simulink model "mavsim_chap4"  (R2022b)
settings: Solver=ode45  StartTime=0.0  StopTime=10000  RelTol=1e-3  EnableMultiTasking=on
InitFcn:
  | addpath('../chap_2')
  | addpath('../../parameters/')
  | aerosonde_parameters
  | simulation_parameters
  | wind_parameters
  | addpath('../chap_3')
  | addpath('../chap_4')
  | addpath('../../tools/')
undefined symbols (not defined in the file or in its folder): drawAircraft, forces_moments, MAV, plotmavstatevariables, SIM, WIND
libraries: simulink x4
settings Model: Creator=beard  LastModifiedBy=william
settings SolverCC: AlgebraicLoopSolver=TrustRegion
settings DataIOCC: LimitDataPoints=on  SaveFormat=Array  SignalLoggingSaveFormat=ModelDataLogs  ReturnWorkspaceOutputs=off
settings OptimizationCC: ExpressionDepthLimit=2147483647  InitFltsAndDblsToZero=on  LifeSpan=inf
settings DebuggingCC: UnderspecifiedInitializationDetection=Classic  MergeDetectMultiDrivingBlocksExec=none  SolverPrmCheckMsg=warning  FcnCallInpInsideContextMsg=warning  UnconnectedInputMsg=warning  UnconnectedOutputMsg=warning  UnconnectedLineMsg=warning  StateNameClashWarn=warning  SFUnexpectedBacktrackingDiag=warning  SFNoUnconditionalDefaultTransitionDiag=warning  SFExecutionAtInitializationDiag=none  SFMachineParentedDataDiag=warning  ArithmeticOperatorsInVariantConditions=warning
settings HardwareCC: ProdBitPerPointer=32  ProdBitPerSizeT=32  ProdBitPerPtrDiffT=32  ProdLargestAtomicFloat=None  ProdIntDivRoundTo=Undefined  ProdEndianess=Unspecified  ProdWordSize=32  ProdHWDeviceType=32-bit Generic
settings ModelReferenceCC: EnableRefExpFcnMdlSchedulingChecks=on  PropagateSignalLabelsOutOfModel=off
settings SFSimCC: SimUseLocalCustomCode=off  CustomCodeUndefinedFunction=UseInterfaceOnly
settings RTWCC: RTWUseLocalCustomCode=off
settings CodeAppCC: StateflowObjectComments=on
settings GRTTargetCC: TargetLangStandard=C89/C90 (ANSI)  CombineOutputUpdateFcns=off  GRTInterface=on
settings ConfigComp: CovMetricSettings=dw  CovSaveCumulativeToWorkspaceVar=on  CovSaveSingleToWorkspaceVar=on  CovExternalEMLEnable=off  CovSFcnEnable=off

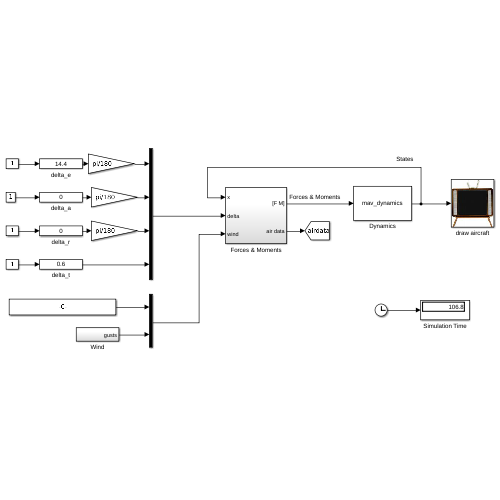
[thumbnail: Simulink's stored preview of the top-level diagram]
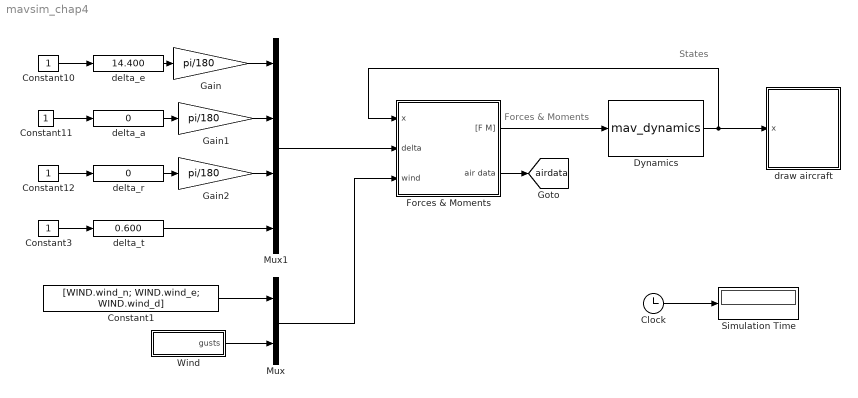
== system mavsim_chap4 ==
  note: Forces & Moments
  note: States
  Clock : Clock
  Constant1 : Constant  Value=[WIND.wind_n; WIND.wind_e; WIND.wind_d]
  Constant{3,10..12} (4 alike) : Constant
  Dynamics : S-Function  FunctionName=mav_dynamics  Parameters=MAV  SFunctionDeploymentMode=off  EnableBusSupport=off
  Forces & Moments : Subsystem
  Gain : Gain  Gain=pi/180
  Gain1 : Gain  Gain=pi/180
  Gain2 : Gain  Gain=pi/180
  Mux : Mux  Inputs=2
  Mux1 : Mux
  Simulation Time : Display
  Wind : Subsystem
  delta_a : simulink/Math Operations/Slider Gain  gain=0  low=-45  high=45
  delta_e : simulink/Math Operations/Slider Gain  gain=14.400  low=-45  high=45
  delta_r : simulink/Math Operations/Slider Gain  gain=0  low=-45  high=45
  delta_t : simulink/Math Operations/Slider Gain  gain=0.600  low=0  high=1
  draw aircraft : Subsystem
      mask Display: image(imread('tv.jpg'))
  tag scope: airdata=global
  wires:
  Constant10/1 -> delta_e/1
  Constant11/1 -> delta_a/1
  Constant12/1 -> delta_r/1
  Dynamics/1 -> draw aircraft/1(x), Forces & Moments/1(x)
  delta_r/1 -> Gain2/1
  delta_a/1 -> Gain1/1
  delta_e/1 -> Gain/1
  Constant3/1 -> delta_t/1
  delta_t/1 -> Mux1/4
  Mux1/1 -> Forces & Moments/2(delta)
  Forces & Moments/1("[F M]") -> Dynamics/1
  Clock/1 -> Simulation Time/1
  Mux/1 -> Forces & Moments/3(wind)
  Wind/1(gusts) -> Mux/2
  Constant1/1 -> Mux/1
  Forces & Moments/2(air data) -> [airdata]
  Gain/1 -> Mux1/1
  Gain1/1 -> Mux1/2
  Gain2/1 -> Mux1/3

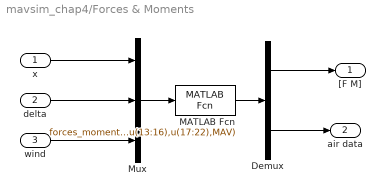
== system mavsim_chap4/Forces & Moments ==
  x : Inport
  delta : Inport  Port=2
  wind : Inport  Port=3
  Demux : Demux  Outputs=[6;6]
  MATLAB Fcn : MATLABFcn  MATLABFcn=forces_moments(u(1:12),u(13:16),u(17:22),MAV)  OutputDimensions=12
  Mux : Mux  Inputs=3
  "[F M]" : Outport  VectorParamsAs1DForOutWhenUnconnected=off
  air data : Outport  Port=2  VectorParamsAs1DForOutWhenUnconnected=off
  wires:
  x/1 -> Mux/1
  delta/1 -> Mux/2
  wind/1 -> Mux/3
  MATLAB Fcn/1 -> Demux/1
  Demux/1 -> "[F M]"/1
  Mux/1 -> MATLAB Fcn/1
  Demux/2 -> air data/1

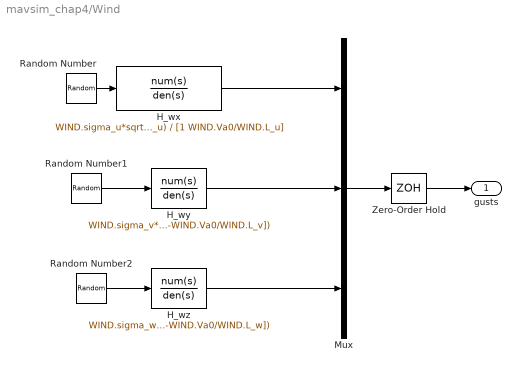
== system mavsim_chap4/Wind ==
  H_wx : TransferFcn  Numerator=WIND.sigma_u*sqrt(2*WIND.Va0/WIND.L_u)  Denominator=[1 WIND.Va0/WIND.L_u]
  H_wy : TransferFcn  Numerator=WIND.sigma_v*sqrt(3*WIND.Va0/WIND.L_v)*[0, 1, WIND.Va0/sqrt(3)/WIND.L_v]  Denominator=poly([-WIND.Va0/WIND.L_v, -WIND.Va0/WIND.L_v])
  H_wz : TransferFcn  Numerator=WIND.sigma_w*sqrt(3*WIND.Va0/WIND.L_w)*[0, 1, WIND.Va0/sqrt(3)/WIND.L_w]  Denominator=poly([-WIND.Va0/WIND.L_w, -WIND.Va0/WIND.L_w])
  Mux : Mux  Inputs=3
  Random Number : RandomNumber  SampleTime=0
  Random Number1 : RandomNumber  SampleTime=0
  Random Number2 : RandomNumber  SampleTime=0
  Zero-Order Hold : ZeroOrderHold  SampleTime=SIM.ts_simulation
  gusts : Outport  VectorParamsAs1DForOutWhenUnconnected=off
  wires:
  H_wx/1 -> Mux/1
  Random Number/1 -> H_wx/1
  H_wy/1 -> Mux/2
  Random Number1/1 -> H_wy/1
  H_wz/1 -> Mux/3
  Random Number2/1 -> H_wz/1
  Mux/1 -> Zero-Order Hold/1
  Zero-Order Hold/1 -> gusts/1

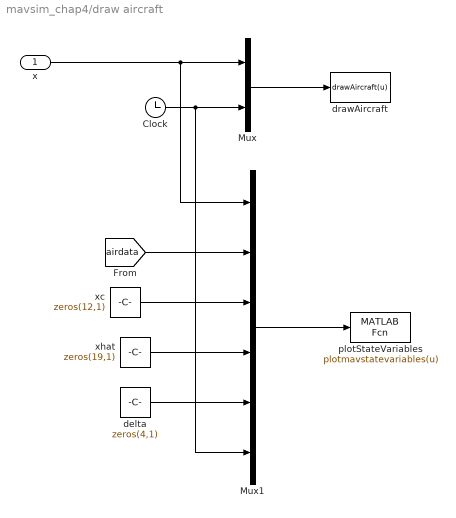
== system mavsim_chap4/draw aircraft ==
  x : Inport
  Clock : Clock
  Mux : Mux  Inputs=2
  Mux1 : Mux  Inputs=6
  delta : Constant  Value=zeros(4,1)
  drawAircraft : MATLABFcn  MATLABFcn=drawAircraft(u)  OutputDimensions=0  SampleTime=0.1
  plotStateVariables : MATLABFcn  MATLABFcn=plotmavstatevariables(u)  OutputDimensions=0  SampleTime=0.1
  xc : Constant  Value=zeros(12,1)
  xhat : Constant  Value=zeros(19,1)
  wires:
  [airdata] -> Mux1/2
  delta/1 -> Mux1/5
  xc/1 -> Mux1/3
  xhat/1 -> Mux1/4
  Mux1/1 -> plotStateVariables/1
  Clock/1 -> Mux1/6, Mux/2
  x/1 -> Mux1/1, Mux/1
  Mux/1 -> drawAircraft/1
